simulink library "rgbled_temp"  (R2024b)
settings: Solver=VariableStepAuto  StartTime=0.0  StopTime=10.0  RelTol=1e-3
settings Model: Creator=mainuser  LastModifiedBy=mainuser

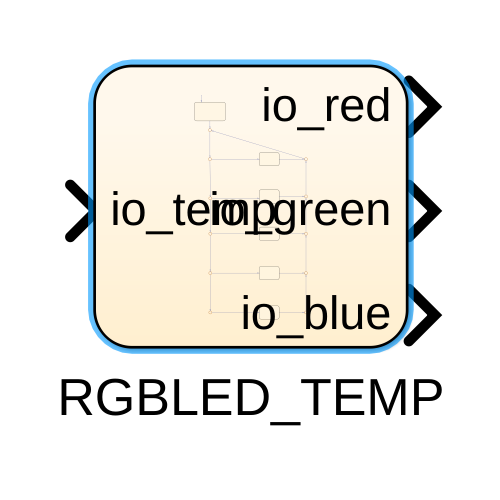
[thumbnail: Simulink's stored preview of the top-level diagram]
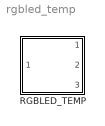
== system rgbled_temp ==
  RGBLED_TEMP : Stateflow chart  TreatAsAtomicUnit=on

== stateflow chart rgbled_temp/RGBLED_TEMP ==
  state Init
    en: io_red=0;
    io_green=0;
    io_blue=0;
  state Blue
    en: io_red=0;
    io_green=0;
    io_blue=100;
  state Violet
    en: io_red=93;
    io_green=51;
    io_blue=93;
  state Yellow
    en: io_red=100;
    io_green=100;
    io_blue=0;
  state Orange
    en: io_red=100;
    io_green=65;
    io_blue=0;
  state Red
    en: io_red=100;
    io_green=0;
    io_blue=0;
  (default) -> Init
  (junction 36) -> Init [order 2]
  Init -> (junction 57)
  (junction 46) -> (junction 57) : [hasChanged(io_temp)]
  (junction 57) -> (junction 17)
  (junction 17) -> Blue [order 1] : [io_temp>=16 && io_temp<=18]
  Blue -> (junction 46)
  (junction 17) -> (junction 25) [order 2]
  (junction 45) -> (junction 46)
  Violet -> (junction 45)
  (junction 25) -> Violet [order 1] : [io_temp>=19 && io_temp<=21]
  (junction 44) -> (junction 45)
  (junction 25) -> (junction 29) [order 2]
  (junction 29) -> Yellow [order 1] : [io_temp>=22 && io_temp<=24]
  Yellow -> (junction 44)
  (junction 29) -> (junction 35) [order 2]
  (junction 43) -> (junction 44)
  (junction 35) -> Orange [order 1] : [io_temp>=25 && io_temp<=27]
  Orange -> (junction 43)
  (junction 35) -> (junction 36) [order 2]
  (junction 42) -> (junction 43)
  Red -> (junction 42)
  (junction 36) -> Red [order 1] : [io_temp>=28 && io_temp<=30]
  data: io_temp input; io_red output; io_green output; io_blue output
